simulink model "feedf"  (Simulink 7.8)
settings: Solver=FixedStepDiscrete  StartTime=0.0  StopTime=2  FixedStep=1/4096  RelTol=1e-3
settings Model: Creator=root  LastModifiedBy=root

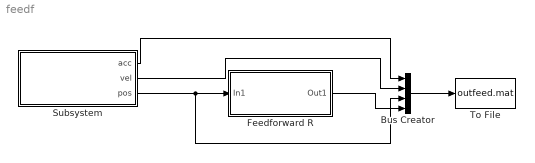
== system feedf ==
  Bus Creator : BusCreator
  Feedforward R : Subsystem
  Subsystem : Subsystem
      settings: OpenFcn=r3g_main
      mask Type: Ref3
      mask Display: disp('Ref3');
  To File : ToFile  Filename=outfeed.mat  MatrixName=out
  wires:
  Subsystem/3(pos) -> Feedforward R/1(In1), Bus Creator/3
  Bus Creator/1 -> To File/1
  Subsystem/1(acc) -> Bus Creator/1
  Subsystem/2(vel) -> Bus Creator/2
  Feedforward R/1(Out1) -> Bus Creator/4

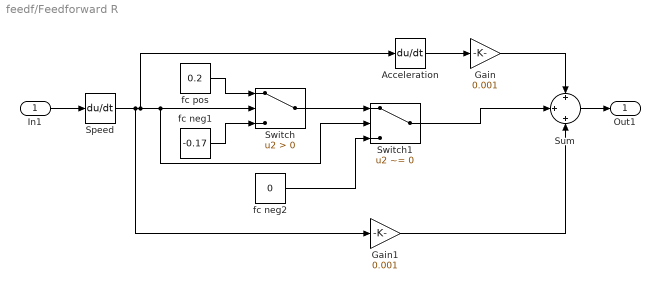
== system feedf/Feedforward R ==
  In1 : Inport
  Acceleration : Derivative
  Gain : Gain  Gain=0.001
  Gain1 : Gain  Gain=0.001
  Speed : Derivative
  Sum : Sum  Inputs=+|+|+
  Switch : Switch  Criteria=u2 > Threshold
  Switch1 : Switch  Criteria=u2 ~= 0
  fc neg1 : Constant  Value=-0.17
  fc neg2 : Constant  Value=0
  fc pos : Constant  Value=0.2
  Out1 : Outport
  wires:
  In1/1 -> Speed/1
  Acceleration/1 -> Gain/1
  Speed/1 -> Acceleration/1, Switch/2, Switch1/2, Gain1/1
  Sum/1 -> Out1/1
  Gain/1 -> Sum/1
  Gain1/1 -> Sum/3
  fc pos/1 -> Switch/1
  fc neg1/1 -> Switch/3
  Switch/1 -> Switch1/1
  fc neg2/1 -> Switch1/3
  Switch1/1 -> Sum/2

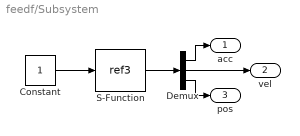
== system feedf/Subsystem ==
  Constant : Constant
  Demux : Demux  Outputs=3
  S-Function : S-Function  FunctionName=ref3  Parameters=ref_part  EnableBusSupport=off
      settings: OpenFcn=global ref_part; r3g_main
  acc : Outport
  vel : Outport  Port=2
  pos : Outport  Port=3
  wires:
  Constant/1 -> S-Function/1
  S-Function/1 -> Demux/1
  Demux/1 -> acc/1
  Demux/2 -> vel/1
  Demux/3 -> pos/1
